simulink model "washout1"  (R2018b)
settings: Solver=VariableStepAuto  StartTime=0.0  StopTime=50  RelTol=1e-3
settings Model: Creator=15705  LastModifiedBy=15705

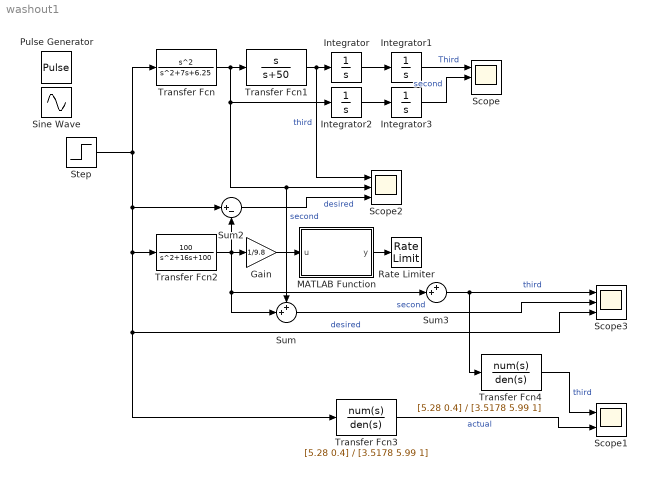
== system washout1 ==
  Gain : Gain  Gain=1/9.8
  Integrator{,1..3} (4 alike) : Integrator
  MATLAB Function : MATLAB Function  TreatAsAtomicUnit=on
  Pulse Generator : DiscretePulseGenerator  PulseType=Time based  Period=10  PulseWidth=50
  Rate Limiter : RateLimiter  RisingSlewLimit=0.0068  FallingSlewLimit=-0.0068  SampleTimeMode=inherited
  Scope : Scope  NumInputPorts=3
  Scope1 : Scope  NumInputPorts=2
  Scope2 : Scope  NumInputPorts=3
  Scope3 : Scope  NumInputPorts=3
  Sine Wave : Sin  Frequency=2  SampleTime=0
  Step : Step  Time=10  Before=1  After=0  SampleTime=0
  Sum : Sum  Inputs=++|
  Sum2 : Sum  Inputs=|+-
  Sum3 : Sum  Inputs=++|
  Transfer Fcn : TransferFcn  Numerator=[1 0 0]  Denominator=[1 7 6.25]
  Transfer Fcn1 : TransferFcn  Numerator=[1 0]  Denominator=[1 50]
  Transfer Fcn2 : TransferFcn  Numerator=[100]  Denominator=[1 16 100]
  Transfer Fcn3 : TransferFcn  Numerator=[5.28 0.4]  Denominator=[3.5178 5.99 1]
  Transfer Fcn4 : TransferFcn  Numerator=[5.28 0.4]  Denominator=[3.5178 5.99 1]
  wires:
  Integrator/1 -> Integrator1/1
  Step/1 -> Transfer Fcn/1, Sum2/1, Scope3/3, Transfer Fcn3/1, Transfer Fcn2/1  "desired"
  Integrator1/1 -> Scope/1  "Third"
  Transfer Fcn/1 -> Sum/1, Scope2/2, Integrator2/1, Transfer Fcn1/1  "second"
  Transfer Fcn1/1 -> Scope2/1, Integrator/1  "third"
  Integrator2/1 -> Integrator3/1
  Integrator3/1 -> Scope/2  "second"
  Transfer Fcn2/1 -> Sum3/2, Sum/2, Sum2/2, Gain/1
  Gain/1 -> MATLAB Function/1(u)
  MATLAB Function/1(y) -> Rate Limiter/1
  Transfer Fcn3/1 -> Scope1/2  "actual"
  Sum2/1 -> Scope2/3  "desired"
  Sum/1 -> Scope3/2  "second"
  Sum3/1 -> Transfer Fcn4/1, Scope3/1  "third"
  Transfer Fcn4/1 -> Scope1/1  "third"

== matlab function washout1/MATLAB Function ==
  data: u input; y output
function y = fcn(u)
y=asin(u);
